simulink model "Identification"  (R2021a)
settings: Solver=ode5  StartTime=0.0  StopTime=t(length(t))  FixedStep=t(2)-t(1)  RelTol=1e-3  EnableMultiTasking=on
settings Model: Creator=LiberT  LastModifiedBy=Maxime
settings SolverCC: AlgebraicLoopSolver=TrustRegion
settings DataIOCC: LimitDataPoints=on  SaveFormat=Array  SignalLoggingSaveFormat=ModelDataLogs  ReturnWorkspaceOutputs=off
settings OptimizationCC: BlockReduction=off  BooleanDataType=off  ExpressionDepthLimit=2147483647  InitFltsAndDblsToZero=on  LifeSpan=inf
settings DebuggingCC: SaveWithParameterizedLinksMsg=none  UnderspecifiedInitializationDetection=Classic  MergeDetectMultiDrivingBlocksExec=none  SignalResolutionControl=TryResolveAllWithWarning  MultiTaskDSMMsg=warning  MultiTaskCondExecSysMsg=none  FcnCallInpInsideContextMsg=warning  StateNameClashWarn=warning  SFUnexpectedBacktrackingDiag=warning  SFNoUnconditionalDefaultTransitionDiag=warning  SFExecutionAtInitializationDiag=none  SFMachineParentedDataDiag=warning  ArithmeticOperatorsInVariantConditions=warning
settings HardwareCC: ProdBitPerPointer=32  ProdBitPerSizeT=32  ProdBitPerPtrDiffT=32  ProdLargestAtomicFloat=None  ProdIntDivRoundTo=Undefined  ProdEndianess=Unspecified  ProdWordSize=32  ProdHWDeviceType=32-bit Generic  TargetUnknown=on
settings ModelReferenceCC: PropagateSignalLabelsOutOfModel=off
settings SFSimCC: SimUseLocalCustomCode=off  CustomCodeUndefinedFunction=UseInterfaceOnly
settings RTWCC: RTWUseLocalCustomCode=off
settings CodeAppCC: StateflowObjectComments=on
settings GRTTargetCC: TargetFcnLib=ansi_tfl_tmw.mat  TargetLangStandard=C89/C90 (ANSI)  ModelReferenceCompliant=off  CompOptLevelCompliant=off  CombineOutputUpdateFcns=off  MatFileLogging=off  GRTInterface=on
settings ConfigComp: CovMetricSettings=dw  CovSaveCumulativeToWorkspaceVar=on  CovSaveSingleToWorkspaceVar=on  CovExternalEMLEnable=off  CovSFcnEnable=off

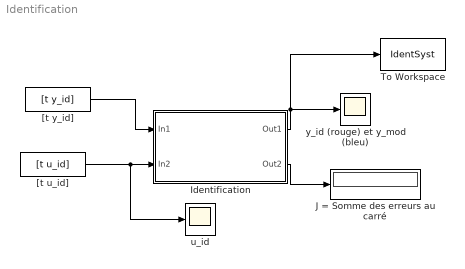
== system Identification ==
  Identification : Subsystem  mask(Identification){num=[1.332], den=[0.2 1], theta=0}
      mask prompts: num "Numérateur"; den "Dénominateur"; theta "Retard"
      mask help: Permet l'identification d'un système linéaire.
      mask Help:
      | Numérateur: Vecteur contenant le numérateur de la fonction de transfert du modèle en puissance décroissante de s. Exemple: [3 4 1] correspond à 3s^2+4s+1.
      | 
      | Dénominateur: Vecteur contenant le dénominateur de la fonction de transfert du modèle en puissance décroissante de s. Le dénominateur doit être d'ordre égal ou supérieur au numérateur.
      | 
      | Retard: Retard de la fonction de transfert du modèle. Il doit être un multiple de la période d'échantillonnage.
      | 
      | 
      | Information sur les ports d'entrée et de sortie (que vous ne devez pas modifier):
      | 
      | - Le port d'entrée #1 du bloc doit recevoir la matrice [t u_id] où t est le vecteur temps et u_id le vecteur entrée du système linéaire auquel on a soustrait le point d'opération. Le vecteur temps doit être à période d'échantillonnage constante.
      | 
      | - Le port d'entrée #2 du bloc doit recevoir la matrice [t y_id] où t est le vecteur temps et y_id le vecteur sortie du système linéaire auquel on a soustrait le point d'opération.
      | 
      | - Le port de sortie #1 du bloc génére une matrice contenant les vecteurs y_id et y_mod (la sortie du modèle). Ce port peut être directement connecté à un oscilloscope pour comparer les deux signaux.
      | 
      | - Le port de sortie #2 du bloc génère le critère J qui est la somme des carrés des différences entre la sortie mesurée et la sortie du modèle.
      mask Display:
      | port_label('input', 1, '[t y_id]')
      | port_label('input', 2, '[t u_id]')
      | port_label('output', 1, 'y_id et y_mod')
      | port_label('output', 2, 'J')
  J = Somme des erreurs au carré : Display
  To Workspace : ToWorkspace  VariableName=IdentSyst  SampleTime=-1
  "[t u_id]" : FromWorkspace  VariableName=[t u_id]  SampleTime=t(2)-t(1)  ZeroCross=off
  "[t y_id]" : FromWorkspace  VariableName=[t y_id]  SampleTime=t(2)-t(1)  ZeroCross=off
  u_id : Scope
  y_id (rouge) et y_mod (bleu) : Scope
  wires:
  Identification/2(Out2) -> J = Somme des erreurs au carré/1
  Identification/1(Out1) -> To Workspace/1, y_id (rouge) et y_mod (bleu)/1
  "[t y_id]"/1 -> Identification/1(In1)
  "[t u_id]"/1 -> Identification/2(In2), u_id/1

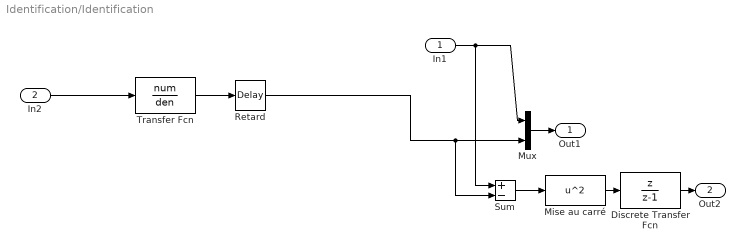
== system Identification/Identification ==
  In1 : Inport
  In2 : Inport  Port=2
  Discrete Transfer Fcn : DiscreteTransferFcn  Numerator=[1 0]  Denominator=[1 -1]  SampleTime=t(2)-t(1)
  Mise au carré : Fcn  Expr=u^2
  Mux : Mux  Inputs=2
  Retard : TransportDelay  DelayTime=theta
  Sum : Sum  Inputs=+-  InputSameDT=on  SaturateOnIntegerOverflow=on  OutDataTypeStr=Inherit: Same as first input
  Transfer Fcn : TransferFcn  Numerator=num  Denominator=den
  Out1 : Outport  VectorParamsAs1DForOutWhenUnconnected=off
  Out2 : Outport  Port=2  VectorParamsAs1DForOutWhenUnconnected=off
  wires:
  Sum/1 -> Mise au carré/1
  Mise au carré/1 -> Discrete Transfer Fcn/1
  Transfer Fcn/1 -> Retard/1
  In1/1 -> Mux/1, Sum/1
  In2/1 -> Transfer Fcn/1
  Mux/1 -> Out1/1
  Discrete Transfer Fcn/1 -> Out2/1
  Retard/1 -> Sum/2, Mux/2
